simulink model "CDR"  (R2020a)
settings: Solver=VariableStepAuto  StartTime=0.0  StopTime=50  MaxStep=1e-3  RelTol=1e-5
libraries: simulink x4
settings Model: Creator=hassa  LastModifiedBy=hassa

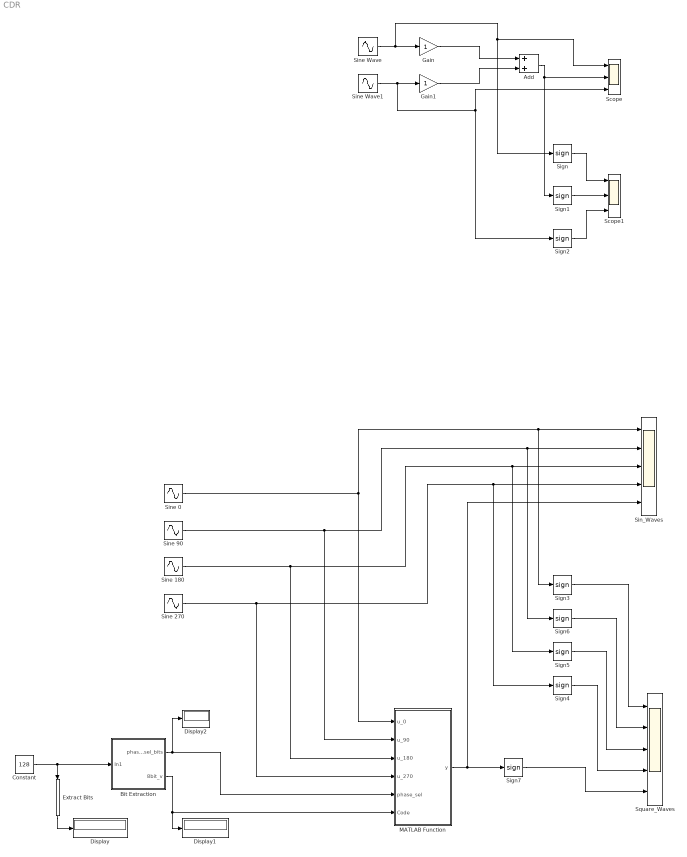
== system CDR ==
  Add : Sum
  Bit Extraction : Subsystem
  Constant : Constant  Value=128  OutDataTypeStr=uint16
  Display : Display
      settings: Format=binary (Stored Integer)
  Display1 : Display
  Display2 : Display
  Extract Bits : simulink/Logic and Bit Operations/Extract Bits  bitsToExtract=Range of bits  numBits=8  bitIdxRange=[0 9]  outScalingMode=Preserve fixed-point scaling
  Gain : Gain
  Gain1 : Gain
  MATLAB Function : MATLAB Function  TreatAsAtomicUnit=on
  Scope : Scope  NumInputPorts=3
  Scope1 : Scope  NumInputPorts=3
  Sign{,1..7} (8 alike) : Signum
  Sin_Waves : Scope  NumInputPorts=5
  Sine 0 : Sin  SampleTime=0
  Sine 180 : Sin  Phase=-pi  SampleTime=0
  Sine 270 : Sin  Phase=(-3*pi)/2  SampleTime=0
  Sine 90 : Sin  Phase=-pi/2  SampleTime=0
  Sine Wave : Sin  SampleTime=0
  Sine Wave1 : Sin  Phase=-pi/2  SampleTime=0
  Square_Waves : Scope  NumInputPorts=5
  wires:
  Sine Wave/1 -> Sign/1, Scope/1, Gain/1
  Sine Wave1/1 -> Sign2/1, Scope/3, Gain1/1
  Gain1/1 -> Add/2
  Gain/1 -> Add/1
  Add/1 -> Sign1/1, Scope/2
  Sign/1 -> Scope1/1
  Sign1/1 -> Scope1/2
  Sign2/1 -> Scope1/3
  Sine 0/1 -> MATLAB Function/1(u_0), Sin_Waves/1, Sign3/1
  Sine 180/1 -> Sign5/1, Sin_Waves/3, MATLAB Function/3(u_180)
  Constant/1 -> Bit Extraction/1(In1), Extract Bits/1
  Bit Extraction/1(phase_sel_bits) -> Display2/1, MATLAB Function/5(phase_sel)
  Bit Extraction/2(8bit_v) -> Display1/1, MATLAB Function/6(Code)
  Extract Bits/1 -> Display/1
  Sine 90/1 -> MATLAB Function/2(u_90), Sign6/1, Sin_Waves/2
  Sine 270/1 -> MATLAB Function/4(u_270), Sign4/1, Sin_Waves/4
  MATLAB Function/1(y) -> Sign7/1, Sin_Waves/5
  Sign3/1 -> Square_Waves/1
  Sign6/1 -> Square_Waves/2
  Sign5/1 -> Square_Waves/3
  Sign4/1 -> Square_Waves/4
  Sign7/1 -> Square_Waves/5

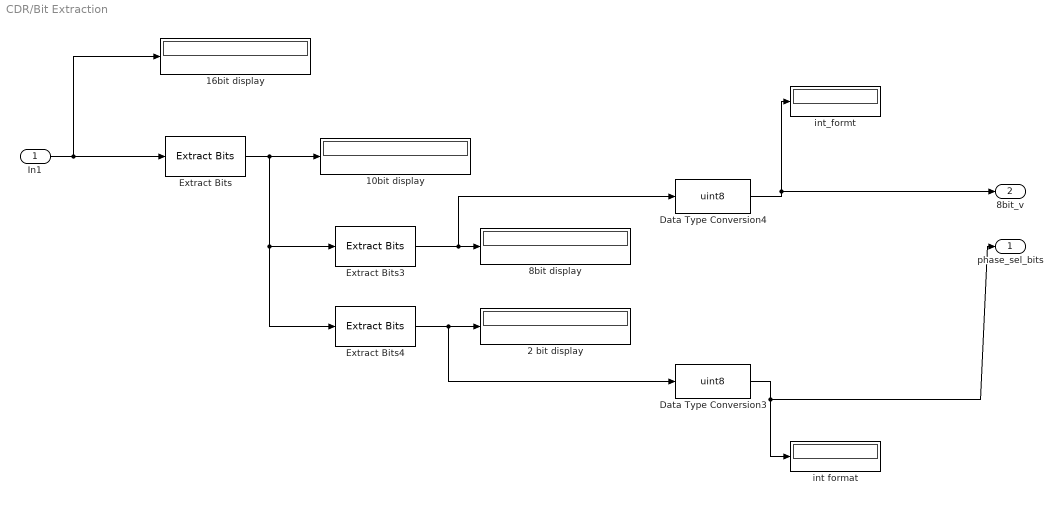
== system CDR/Bit Extraction ==
  In1 : Inport
  10bit display : Display
      settings: Format=binary (Stored Integer)
  16bit display : Display
      settings: Format=binary (Stored Integer)
  2 bit display : Display
      settings: Format=binary (Stored Integer)
  8bit display : Display
      settings: Format=binary (Stored Integer)
  Data Type Conversion3 : DataTypeConversion  OutDataTypeStr=uint8
  Data Type Conversion4 : DataTypeConversion  OutDataTypeStr=uint8
  Extract Bits : simulink/Logic and Bit Operations/Extract Bits  bitsToExtract=Range of bits  numBits=8  bitIdxRange=[0 9]  outScalingMode=Preserve fixed-point scaling
  Extract Bits3 : simulink/Logic and Bit Operations/Extract Bits  bitsToExtract=Range of bits  numBits=8  bitIdxRange=[0 7]  outScalingMode=Preserve fixed-point scaling
  Extract Bits4 : simulink/Logic and Bit Operations/Extract Bits  bitsToExtract=Range of bits  numBits=8  bitIdxRange=[8 9]  outScalingMode=Treat bit field as an integer
  int format : Display
  int_formt : Display
  phase_sel_bits : Outport  VectorParamsAs1DForOutWhenUnconnected=off
  8bit_v : Outport  Port=2
  wires:
  In1/1 -> Extract Bits/1, 16bit display/1
  Extract Bits4/1 -> Data Type Conversion3/1, 2 bit display/1
  Extract Bits3/1 -> Data Type Conversion4/1, 8bit display/1
  Extract Bits/1 -> Extract Bits4/1, Extract Bits3/1, 10bit display/1
  Data Type Conversion3/1 -> int format/1, phase_sel_bits/1
  Data Type Conversion4/1 -> 8bit_v/1, int_formt/1

== matlab function CDR/MATLAB Function ==
  data: u_0 input; y output; u_90 input; u_180 input; u_270 input; phase_sel input; Code input
function y  = fcn(u_0, u_90, u_180, u_270, phase_sel, Code)

if phase_sel == 0
    p1 = u_0;
    p2 = u_90;
elseif phase_sel == 1
    p1 = u_90;
    p2 = u_180;        
elseif phase_sel == 2
    p1 = u_180;
    p2 = u_270; 
else
    p1 = u_270;
    p2 = u_0;    
end



x1 = (double(Code) / 255.0 );  % Corrected the computation of x1
x2 = (1.0 - x1);  % Corrected the computation of x2

disp(Code)

%disp(x1)
%disp(x2)

y = x1 * p2 + x2 * p1 ;
%y = x1 * p2 + x2 * p1;
